simulink model "bus_simple"  (Simulink 8.0)
settings: Solver=ode45  StartTime=0.0  StopTime=10.0  RelTol=1e-3
settings Model: Creator=massif  LastModifiedBy=massif

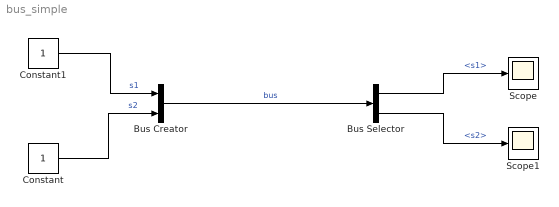
== system bus_simple ==
  Bus Creator : BusCreator  Inputs=2
  Bus Selector : BusSelector  OutputSignals=s1,s2
  Constant : Constant
  Constant1 : Constant
  Scope : Scope
  Scope1 : Scope
  wires:
  Constant1/1 -> Bus Creator/1  "s1"
  Bus Creator/1 -> Bus Selector/1  "bus"
  Bus Selector/1 -> Scope/1  "<s1>"
  Bus Selector/2 -> Scope1/1  "<s2>"
  Constant/1 -> Bus Creator/2  "s2"
